simulink model "mymodel"  (R2013a)
settings: Solver=ode45  StartTime=0.0  StopTime=10.0  RelTol=1e-3
libraries: cstblocks x1
settings Model: Creator=ugurm  LastModifiedBy=ugurm

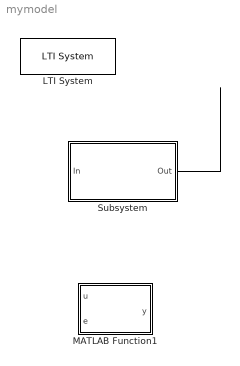
== system mymodel ==
  LTI System : cstblocks/LTI System  sys=tf(1,[1 1])  IC=[]
  MATLAB Function1 : MATLAB Function  TreatAsAtomicUnit=on
  Subsystem : Subsystem
  wires:
  ? -> Subsystem/1(In)
  Subsystem/1(Out) -> ?

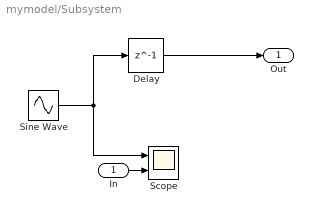
== system mymodel/Subsystem ==
  In : Inport
  Delay : Delay  DelayLength=1  InitialCondition=0
  Scope : Scope  NumInputPorts=2
      settings: YMin=-5~-5  YMax=5~5
  Sine Wave : Sin  SampleTime=0
  Out : Outport
  wires:
  Delay/1 -> Out/1
  Sine Wave/1 -> Delay/1, Scope/1
  In/1 -> Scope/2

== matlab function mymodel/MATLAB Function1 ==
  data: u input; y output; e input
function y = fcn(u,e)
%#codegen

y = u;
